simulink model "car2nd"  (R2021b)
settings: Solver=VariableStepAuto  StartTime=0.0  StopTime=30  RelTol=1e-3
libraries: simulink x1
settings Model: Creator=minna  LastModifiedBy=minna

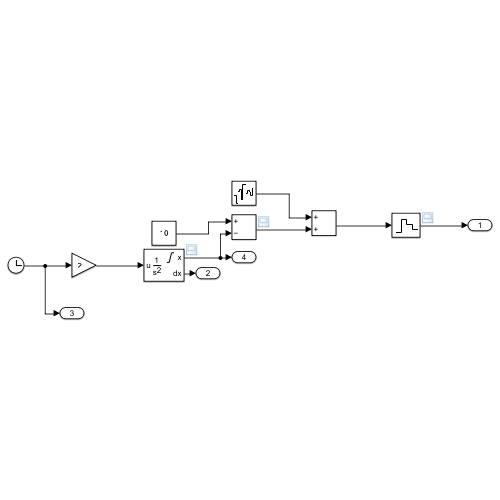
[thumbnail: Simulink's stored preview of the top-level diagram]
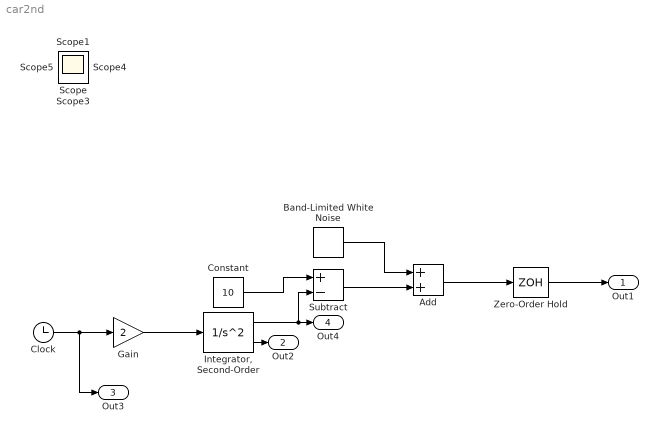
== system car2nd ==
  Add : Sum
  Band-Limited White Noise : simulink/Sources/Band-Limited White Noise  Cov=0.001  Ts=0.1  seed=[23341]
  Clock : Clock
  Constant : Constant  Value=10
  Gain : Gain  Gain=2
  "Integrator, Second-Order" : SecondOrderIntegrator  LimitX=on  UpperLimitX=10
  Subtract : Sum  Inputs=+-
  Zero-Order Hold : ZeroOrderHold  SampleTime=0.1
  Out1 : Outport
  Out2 : Outport  Port=2
  Out3 : Outport  Port=3
  Out4 : Outport  Port=4
  Scope{,1,3..5} (5 alike) : Scope
  wires:
  Gain/1 -> "Integrator, Second-Order"/1
  "Integrator, Second-Order"/2 -> Out2/1
  Clock/1 -> Out3/1, Gain/1
  "Integrator, Second-Order"/1 -> Subtract/2, Out4/1
  Subtract/1 -> Add/2
  Band-Limited White Noise/1 -> Add/1
  Add/1 -> Zero-Order Hold/1
  Zero-Order Hold/1 -> Out1/1
  Constant/1 -> Subtract/1
